simulink model "backup"  (R2014a)
settings: Solver=ode45  StartTime=0.0  StopTime=10.0  RelTol=1e-3
values from neighbouring files (symbols this model uses):
  d = 0.235    [head.m]
libraries: simulink x1
settings Model: Creator=WXY  LastModifiedBy=WXY

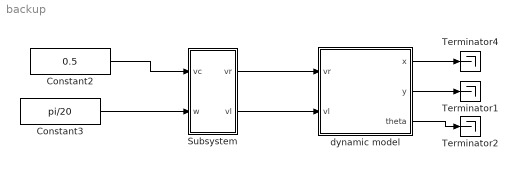
== system backup ==
  Constant2 : Constant  Value=0.5
  Constant3 : Constant  Value=pi/20
  Subsystem : Subsystem
  Terminator1 : Terminator
  Terminator2 : Terminator
  Terminator4 : Terminator
  dynamic model : Subsystem
  wires:
  Subsystem/1(vr) -> dynamic model/1(vr)
  Subsystem/2(vl) -> dynamic model/2(vl)
  Constant3/1 -> Subsystem/2(w)
  Constant2/1 -> Subsystem/1(vc)
  dynamic model/1(x) -> Terminator4/1
  dynamic model/2(y) -> Terminator1/1
  dynamic model/3(theta) -> Terminator2/1

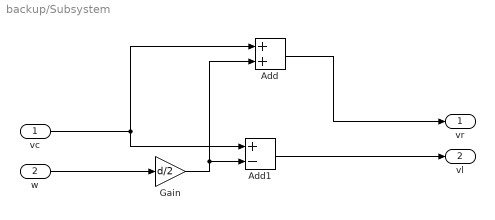
== system backup/Subsystem ==
  vc : Inport
  w : Inport  Port=2
  Add : Sum
  Add1 : Sum  Inputs=+-
  Gain : Gain  Gain=d/2
  vr : Outport
  vl : Outport  Port=2
  wires:
  vc/1 -> Add/1, Add1/1
  w/1 -> Gain/1
  Gain/1 -> Add/2, Add1/2
  Add/1 -> vr/1
  Add1/1 -> vl/1

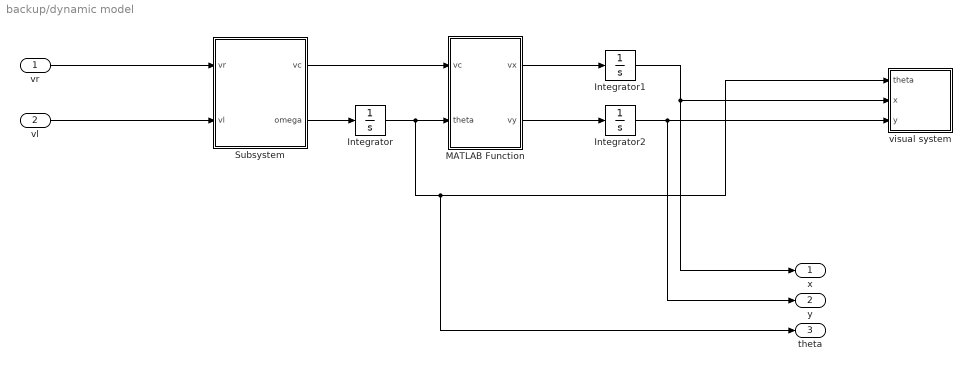
== system backup/dynamic model ==
  vr : Inport
  vl : Inport  Port=2
  Integrator : Integrator
  Integrator1 : Integrator
  Integrator2 : Integrator
  MATLAB Function : MATLAB Function  TreatAsAtomicUnit=on
  Subsystem : Subsystem
  visual system : Subsystem
  x : Outport
  y : Outport  Port=2
  theta : Outport  Port=3
  wires:
  MATLAB Function/2(vy) -> Integrator2/1
  MATLAB Function/1(vx) -> Integrator1/1
  vr/1 -> Subsystem/1(vr)
  vl/1 -> Subsystem/2(vl)
  Subsystem/1(vc) -> MATLAB Function/1(vc)
  Subsystem/2(omega) -> Integrator/1
  Integrator/1 -> theta/1, visual system/1(theta), MATLAB Function/2(theta)
  Integrator1/1 -> x/1, visual system/2(x)
  Integrator2/1 -> y/1, visual system/3(y)

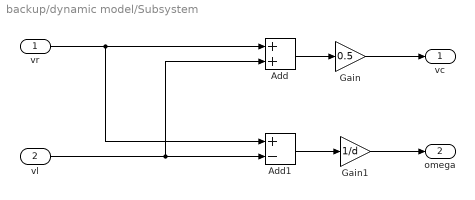
== system backup/dynamic model/Subsystem ==
  vr : Inport
  vl : Inport  Port=2
  Add : Sum
  Add1 : Sum  Inputs=+-
  Gain : Gain  Gain=0.5
  Gain1 : Gain  Gain=1/d
  vc : Outport
  omega : Outport  Port=2
  wires:
  vl/1 -> Add1/2, Add/2
  Gain/1 -> vc/1
  Add1/1 -> Gain1/1
  Add/1 -> Gain/1
  Gain1/1 -> omega/1
  vr/1 -> Add1/1, Add/1

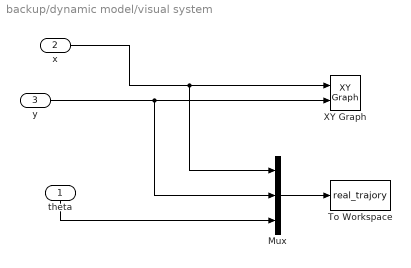
== system backup/dynamic model/visual system ==
  theta : Inport
  x : Inport  Port=2
  y : Inport  Port=3
  Mux : Mux  Inputs=3
  To Workspace : ToWorkspace  VariableName=real_trajory  SaveFormat=Structure With Time  SampleTime=-1
  XY Graph : simulink/Sinks/XY Graph  xmin=-10  xmax=10  ymin=-10  ymax=10  st=-1
  wires:
  Mux/1 -> To Workspace/1
  theta/1 -> Mux/3
  x/1 -> Mux/1, XY Graph/1
  y/1 -> Mux/2, XY Graph/2

== matlab function backup/dynamic model/MATLAB Function ==
  data: vc input; vx output; theta input; vy output
function [vx,vy] = fcn(vc,theta)
%#codegen

vx=vc*cos(theta);
vy=vc*sin(theta);

end
